simulink model "xyxy_sim"  (R2019a)
settings: Solver=VariableStepAuto  StartTime=0.0  StopTime=10.0  RelTol=1e-3
libraries: simulink x2
settings Model: Creator=hanabusa  LastModifiedBy=hanabusa

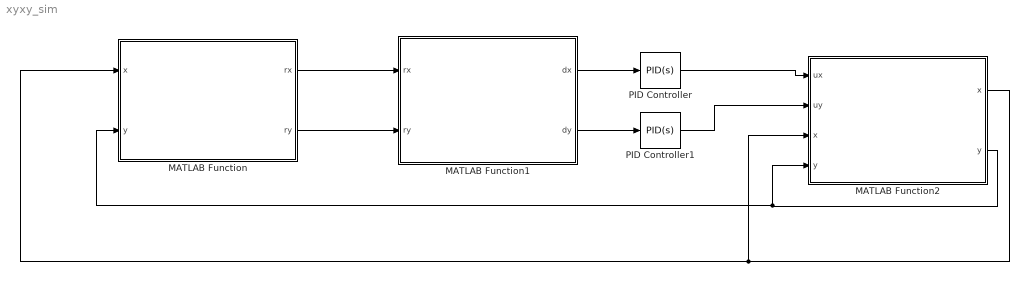
== system xyxy_sim ==
  MATLAB Function : MATLAB Function  TreatAsAtomicUnit=on
  MATLAB Function1 : MATLAB Function  TreatAsAtomicUnit=on
  MATLAB Function2 : MATLAB Function  TreatAsAtomicUnit=on
  PID Controller : simulink/Continuous/PID Controller  Controller=PID  Form=Parallel  TimeDomain=Continuous-time  SampleTime=-1  IntegratorMethod=Forward Euler  FilterMethod=Forward Euler  ControllerParametersSource=internal  P=1  I=1  D=0  UseFilter=on  N=100  TunerSelectOption=Transfer Function Based (PID Tuner App)  InitialConditionSource=internal  InitialConditionForIntegrator=0  InitialConditionForFilter=0  DifferentiatorICPrevScaledInput=0  ExternalReset=none  TrackingMode=off  Kt=1  LimitOutput=off  UpperSaturationLimit=inf  LowerSaturationLimit=-inf  LinearizeAsGain=on  AntiWindupMode=none  Kb=1  POutMin=[]  POutMax=[]  IOutMin=[]  IOutMax=[]  DOutMin=[]  DOutMax=[]  NOutMin=[]  NOutMax=[]  SumOutMin=[]  SumOutMax=[]  SaturationOutMin=[]  SaturationOutMax=[]  PParamMin=[]  PParamMax=[]  IParamMin=[]  IParamMax=[]  DParamMin=[]  DParamMax=[]  NParamMin=[]  NParamMax=[]  KbParamMin=[]  KbParamMax=[]  KtParamMin=[]  KtParamMax=[]  KbOutMin=[]  KbOutMax=[]  KtOutMin=[]  KtOutMax=[]  IntegratorOutMin=[]  IntegratorOutMax=[]  FilterOutMin=[]  FilterOutMax=[]  SumI1OutMin=[]  SumI1OutMax=[]  SumI2OutMin=[]  SumI2OutMax=[]  SumI3OutMin=[]  SumI3OutMax=[]  SumI4OutMin=[]  SumI4OutMax=[]  SumDOutMin=[]  SumDOutMax=[]  DifferentiatorOutMin=[]  DifferentiatorOutMax=[]  FilterDiffOutCoefMin=[]  FilterDiffOutCoefMax=[]  ReciprocalOutMin=[]  ReciprocalOutMax=[]  SumDenOutMin=[]  SumDenOutMax=[]  SumNumOutMin=[]  SumNumOutMax=[]  DivideOutMin=[]  DivideOutMax=[]  IntegratorContinuousStateAttributes=''  IntegratorStateMustResolveToSignalObject=off  IntegratorRTWStateStorageClass=Auto  FilterContinuousStateAttributes=''  FilterStateMustResolveToSignalObject=off  FilterRTWStateStorageClass=Auto  ParallelPVariant=InternalParameters  IdealPVariant=Disabled  IVariant=InternalParameters  DVariant=InternalParameters  IntegratorVariant=Continuous  SatVariant=Disabled  AWVariant=Passthrough  PCopyVariant=Disabled  TRVariant=Disabled  FdbkBlocksVariant=Forward  IdealPFdbkVariant=Disabled  SatFdbkVariant=Disabled  DerivativeFilterVariant=ContFilter  NVariant=InternalParameters  NCopyVariant=Disabled  FilterICVariant=InternalICsFilter  IntegratorICVariant=InternalICs  ExternalResetVariant=Disabled  TRSumVariant=Passthrough  SumFdbkVariant=Disabled  SumVariant=Sum_PID
  PID Controller1 : simulink/Continuous/PID Controller  Controller=PID  Form=Parallel  TimeDomain=Continuous-time  SampleTime=-1  IntegratorMethod=Forward Euler  FilterMethod=Forward Euler  ControllerParametersSource=internal  P=1  I=1  D=0  UseFilter=on  N=100  TunerSelectOption=Transfer Function Based (PID Tuner App)  InitialConditionSource=internal  InitialConditionForIntegrator=0  InitialConditionForFilter=0  DifferentiatorICPrevScaledInput=0  ExternalReset=none  TrackingMode=off  Kt=1  LimitOutput=off  UpperSaturationLimit=inf  LowerSaturationLimit=-inf  LinearizeAsGain=on  AntiWindupMode=none  Kb=1  POutMin=[]  POutMax=[]  IOutMin=[]  IOutMax=[]  DOutMin=[]  DOutMax=[]  NOutMin=[]  NOutMax=[]  SumOutMin=[]  SumOutMax=[]  SaturationOutMin=[]  SaturationOutMax=[]  PParamMin=[]  PParamMax=[]  IParamMin=[]  IParamMax=[]  DParamMin=[]  DParamMax=[]  NParamMin=[]  NParamMax=[]  KbParamMin=[]  KbParamMax=[]  KtParamMin=[]  KtParamMax=[]  KbOutMin=[]  KbOutMax=[]  KtOutMin=[]  KtOutMax=[]  IntegratorOutMin=[]  IntegratorOutMax=[]  FilterOutMin=[]  FilterOutMax=[]  SumI1OutMin=[]  SumI1OutMax=[]  SumI2OutMin=[]  SumI2OutMax=[]  SumI3OutMin=[]  SumI3OutMax=[]  SumI4OutMin=[]  SumI4OutMax=[]  SumDOutMin=[]  SumDOutMax=[]  DifferentiatorOutMin=[]  DifferentiatorOutMax=[]  FilterDiffOutCoefMin=[]  FilterDiffOutCoefMax=[]  ReciprocalOutMin=[]  ReciprocalOutMax=[]  SumDenOutMin=[]  SumDenOutMax=[]  SumNumOutMin=[]  SumNumOutMax=[]  DivideOutMin=[]  DivideOutMax=[]  IntegratorContinuousStateAttributes=''  IntegratorStateMustResolveToSignalObject=off  IntegratorRTWStateStorageClass=Auto  FilterContinuousStateAttributes=''  FilterStateMustResolveToSignalObject=off  FilterRTWStateStorageClass=Auto  ParallelPVariant=InternalParameters  IdealPVariant=Disabled  IVariant=InternalParameters  DVariant=InternalParameters  IntegratorVariant=Continuous  SatVariant=Disabled  AWVariant=Passthrough  PCopyVariant=Disabled  TRVariant=Disabled  FdbkBlocksVariant=Forward  IdealPFdbkVariant=Disabled  SatFdbkVariant=Disabled  DerivativeFilterVariant=ContFilter  NVariant=InternalParameters  NCopyVariant=Disabled  FilterICVariant=InternalICsFilter  IntegratorICVariant=InternalICs  ExternalResetVariant=Disabled  TRSumVariant=Passthrough  SumFdbkVariant=Disabled  SumVariant=Sum_PID
  wires:
  MATLAB Function/1(rx) -> MATLAB Function1/1(rx)
  MATLAB Function/2(ry) -> MATLAB Function1/2(ry)
  MATLAB Function1/1(dx) -> PID Controller/1
  MATLAB Function1/2(dy) -> PID Controller1/1
  PID Controller/1 -> MATLAB Function2/1(ux)
  PID Controller1/1 -> MATLAB Function2/2(uy)
  MATLAB Function2/1(x) -> MATLAB Function/1(x), MATLAB Function2/3("x ")
  MATLAB Function2/2(y) -> MATLAB Function/2(y), MATLAB Function2/4("y ")

== matlab function xyxy_sim/MATLAB Function1 ==
  data: dx output; rx input; dy output; ry input
function [dx,dy]=dxdy3(rx,ry)
N=5;
% desired state
dp21=[-60 0];
dp31=[-30*sqrt(3) 30];
dp32=[-30*sqrt(3) -30];
dp41=[-30*sqrt(3) -30];
dp43=[0 -60];
dp51=[-60 0];
dp54=[-30 -30*sqrt(3)];

dd=zeros(N,N); %目標の相対距離
for i=2:N    
  dd=[0 0 0 0 0;
      norm(dp21) 0 0 0 0;
      norm(dp31) norm(dp32) 0 0 0;
      norm(dp41) 0 norm(dp43) 0 0;
      norm(dp51) 0 0 norm(dp54) 0];
end
dx=zeros(1,N);    %目標位置
dy=zeros(1,N);
sgn=1; %目標の隣接順序 符号を変えれば反転する
%%
 dx(2)=rx(2,1)+dd(2,1);
 dy(2)=ry(2,1);

 for i=2:N-1 %i+1が子．その隣接する点は１とi
        % 隣接点が同じ位置
        if sqrt((rx(i+1,i)-rx(i+1,1))^2+(ry(i+1,i)-ry(i+1,1))^2)==0    
            dx(i+1)=rx(i+1,i)+dd(i+1,i);
            dy(i+1);
        end
        
        % 隣接点が近すぎる
        if 0<sqrt((rx(i+1,i)-rx(i+1,1))^2+(ry(i+1,i)-ry(i+1,1))^2)&&sqrt((rx(i+1,i)-rx(i+1,1))^2+(ry(i+1,i)-ry(i+1,1))^2)<abs(dd(i+1,1)-dd(i+1,i))
            dx(i+1)=rx(i+1,i)-dd(i+1,i)*(rx(i+1,1)-rx(i+1,i))/sqrt((rx(i+1,i)-rx(i+1,1))^2+(ry(i+1,i)-ry(i+1,1))^2);
            dy(i+1)=ry(i+1,i)-dd(i+1,i)*(ry(i+1,1)-ry(i+1,i))/sqrt((rx(i+1,i)-rx(i+1,1))^2+(ry(i+1,i)-ry(i+1,1))^2);
        end
        
        % 好位置
         if abs(dd(i+1,1)-dd(i+1,i))<=sqrt((rx(i+1,i)-rx(i+1,1))^2+(ry(i+1,i)-ry(i+1,1))^2)&&sqrt((rx(i+1,i)-rx(i+1,1))^2+(ry(i+1,i)-ry(i+1,1))^2)<=abs(dd(i+1,1)+dd(i+1,i))
             costheta=(dd(i+1,i)^2+((rx(i+1,i)-rx(i+1,1))^2+(ry(i+1,i)-ry(i+1,1))^2)-dd(i+1,1)^2)/(2*dd(i+1,i)*sqrt((rx(i+1,i)-rx(i+1,1))^2+(ry(i+1,i)-ry(i+1,1))^2));
             sintheta=sqrt(1-costheta^2);
             R=[costheta sgn*sintheta; -sgn*sintheta costheta]; %回転行列
             dx(i+1)=rx(i+1,i)+(R(1,1)*(rx(i+1,1)-rx(i+1,i))+R(1,2)*(ry(i+1,1)-ry(i+1,i)))*dd(i+1,i)/(sqrt((rx(i+1,i)-rx(i+1,1))^2+(ry(i+1,i)-ry(i+1,1))^2));
             dy(i+1)=ry(i+1,i)+(R(2,1)*(rx(i+1,1)-rx(i+1,i))+R(2,2)*(ry(i+1,1)-ry(i+1,i)))*dd(i+1,i)/(sqrt((rx(i+1,i)-rx(i+1,1))^2+(ry(i+1,i)-ry(i+1,1))^2));
         end
         
        % 隣接点が遠すぎる
         if abs(dd(i+1,1)+dd(i+1,i))<sqrt((rx(i+1,i)-rx(i+1,1))^2+(ry(i+1,i)-ry(i+1,1))^2)
             dx(i+1)=rx(i+1,i)+dd(i+1,i)*(rx(i+1,1)-rx(i+1,i))/(sqrt((rx(i+1,i)-rx(i+1,1))^2+(ry(i+1,i)-ry(i+1,1))^2));
             dy(i+1)=ry(i+1,i)+dd(i+1,i)*(ry(i+1,1)-ry(i+1,i))/(sqrt((rx(i+1,i)-rx(i+1,1))^2+(ry(i+1,i)-ry(i+1,1))^2));
         end
 end
end

== matlab function xyxy_sim/MATLAB Function ==
  data: x input; rx output; y input; ry output
function [rx,ry]=relative_position(x,y)
theta=[pi/2 pi/3 -pi/4 2*pi/3 pi];
N=5;
rx=zeros(N,N);   %相対位置　行が基準  
ry=zeros(N,N);

 for i=1:N
     for j=1:N
       rx(i,j)=cos(theta(i))*(x(j)-x(i))+sin(theta(i))*(y(j)-y(i)); %iから見たjの相対位置
       ry(i,j)=-sin(theta(i))*(x(j)-x(i))+cos(theta(i))*(y(j)-y(i));
     end
 end
end

== matlab function xyxy_sim/MATLAB Function2 ==
  data: ux input; uy input; x input; y input; x output; y output
function [x,y]=xyxy(ux,uy,x,y)
theta=[pi/2 pi/3 -pi/4 2*pi/3 pi];
    for i=1:5
    x(i)=x(i)+(ux(i)*cos(theta(i))-uy(i)*sin(theta(i)))*tt;
    y(i)=y(i)+(ux(i)*sin(theta(i))+uy(i)*cos(theta(i)))*tt;
    end
end
